simulink model "ConsolidatedModelV4"  (R2022a)
settings: Solver=ode23t  StartTime=0.0  StopTime=Tf  RelTol=1e-2
undefined symbols (not defined in the file or in its folder): s0
libraries: rllib x3
settings Model: Creator=The MathWorks, Inc.  LastModifiedBy=yangz
settings SolverCC: AlgebraicLoopSolver=TrustRegion
settings DebuggingCC: UnconnectedInputMsg=warning  UnconnectedOutputMsg=warning  UnconnectedLineMsg=warning  SFMachineParentedDataDiag=warning
settings RTWCC: DLArmComputeVersion=19.05

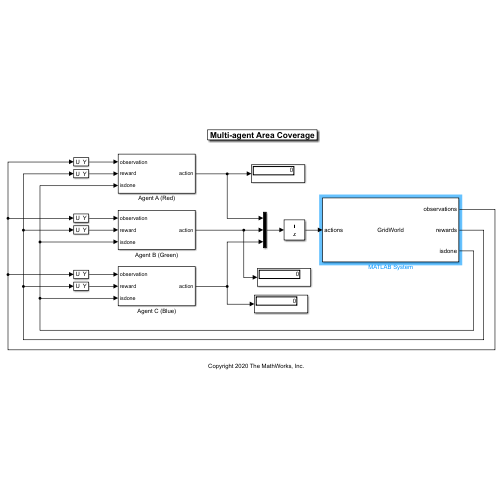
[thumbnail: Simulink's stored preview of the top-level diagram]
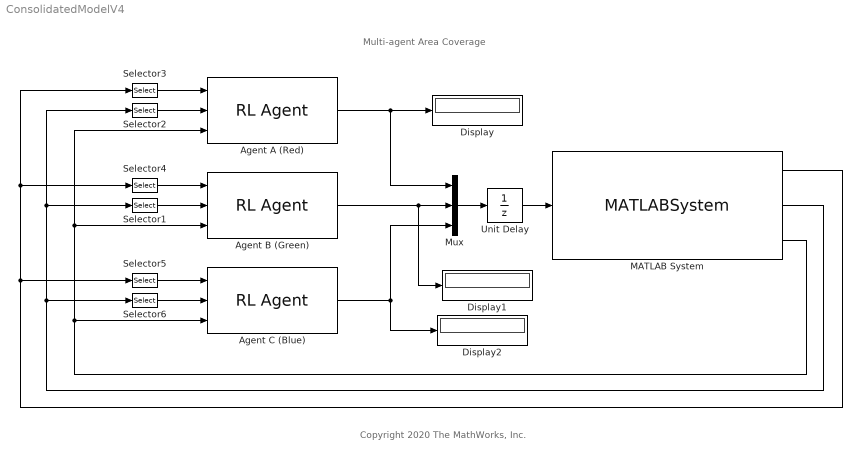
== system ConsolidatedModelV4 ==
  note: Copyright 2020 The MathWorks, Inc.
  note: Multi-agent Area Coverage
  Agent A (Red) : rllib/RL Agent  Agent=agentA  ExternalActionAsInput=off  ProvideLastAction=off  ProvideCumRwd=off  TreatAsDirectFeedthrough=on  UseStrictObservationDataTypes=off
  Agent B (Green) : rllib/RL Agent  Agent=agentB  ExternalActionAsInput=off  ProvideLastAction=off  ProvideCumRwd=off  TreatAsDirectFeedthrough=on  UseStrictObservationDataTypes=off
  Agent C (Blue) : rllib/RL Agent  Agent=agentC  ExternalActionAsInput=off  ProvideLastAction=off  ProvideCumRwd=off  TreatAsDirectFeedthrough=on  UseStrictObservationDataTypes=off
  Display : Display
  Display1 : Display
  Display2 : Display
  MATLAB System : MATLABSystem  System=GridWorld  InitialStates=s0  Obstacles=obsMat  MaxStepCount=maxsteps  SimulateUsing=Interpreted execution
      mask Type: GridWorld
      mask Display:
      | disp('GridWorld');
      | port_label('input',1,'actions');
      | port_label('output',1,'observations');
      | port_label('output',2,'rewards');
      | port_label('output',3,'isdone');
  Mux : Mux  Inputs=3
  Selector1 : Selector  InputPortWidth=3  IndexOptions=Index vector (dialog)  Indices=2  OutputSizes=1
  Selector2 : Selector  InputPortWidth=3  IndexOptions=Index vector (dialog)  Indices=1  OutputSizes=1
  Selector3 : Selector  NumberOfDimensions=4  InputPortWidth=3  IndexOptions=Select all,Select all,Select all,Index vector (dialog)  Indices=1,1,1,1  OutputSizes=1,1,1,1
  Selector4 : Selector  NumberOfDimensions=4  InputPortWidth=3  IndexOptions=Select all,Select all,Select all,Index vector (dialog)  Indices=1,1,1,2  OutputSizes=1,1,1,1
  Selector5 : Selector  NumberOfDimensions=4  InputPortWidth=3  IndexOptions=Select all,Select all,Select all,Index vector (dialog)  Indices=1,1,1,3  OutputSizes=1,1,1,1
  Selector6 : Selector  InputPortWidth=3  IndexOptions=Index vector (dialog)  Indices=3  OutputSizes=1
  Unit Delay : UnitDelay  SampleTime=-1  HasFrameUpgradeWarning=on
  wires:
  Mux/1 -> Unit Delay/1
  Unit Delay/1 -> MATLAB System/1
  Agent B (Green)/1 -> Mux/2, Display1/1
  Agent A (Red)/1 -> Display/1, Mux/1
  Selector3/1 -> Agent A (Red)/1
  Selector2/1 -> Agent A (Red)/2
  MATLAB System/1 -> Selector3/1, Selector4/1, Selector5/1
  MATLAB System/2 -> Selector6/1, Selector1/1, Selector2/1
  MATLAB System/3 -> Agent C (Blue)/3, Agent B (Green)/3, Agent A (Red)/3
  Selector1/1 -> Agent B (Green)/2
  Selector4/1 -> Agent B (Green)/1
  Agent C (Blue)/1 -> Mux/3, Display2/1
  Selector5/1 -> Agent C (Blue)/1
  Selector6/1 -> Agent C (Blue)/2
